simulink model "ekf2sim_example"  (R2014a)
settings: Solver=FixedStepDiscrete  StartTime=0  StopTime=200  RelTol=1e-3
settings Model: Creator=gcampa  LastModifiedBy=gcampa
settings DataIOCC: LimitDataPoints=off  SignalLoggingSaveFormat=ModelDataLogs  SaveOutput=off  SaveTime=off
settings OptimizationCC: BlockReduction=off  BooleanDataType=off  ExpressionDepthLimit=2147483647  InitFltsAndDblsToZero=on
settings DebuggingCC: SaveWithParameterizedLinksMsg=none  UnderspecifiedInitializationDetection=Classic  SignalResolutionControl=TryResolveAllWithWarning  SolverPrmCheckMsg=none  MultiTaskDSMMsg=warning  MultiTaskCondExecSysMsg=none  FcnCallInpInsideContextMsg=UseLocalSettings  StateNameClashWarn=warning
settings HardwareCC: TargetLongLongMode=on  TargetIntDivRoundTo=Zero  TargetEndianess=LittleEndian  TargetHWDeviceType=MATLAB Host  ProdEqTarget=off
settings RTWCC: IncludeERTFirstTime=on  RTWCompilerOptimization=On
settings GRTTargetCC: TargetFcnLib=ansi_tfl_tmw.mat  CombineOutputUpdateFcns=off  GRTInterface=on

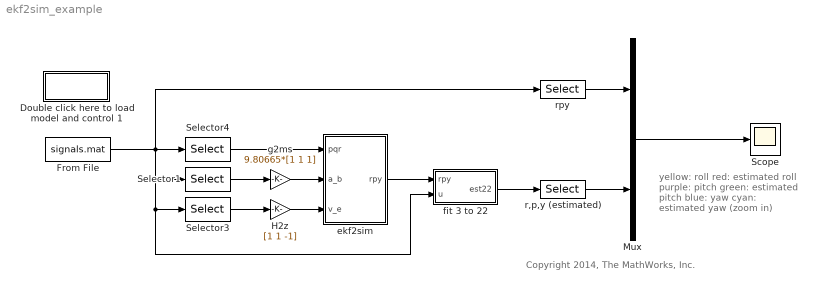
== system ekf2sim_example ==
  note: Copyright 2014, The MathWorks, Inc.
  note: yellow: roll
      | red: estimated roll
      | purple: pitch
      | green: estimated pitch
      | blue: yaw
      | cyan: estimated yaw
      | (zoom in)
  Double click here to load model and control 1 : Subsystem
      mask Display: disp('Measured \nSignals')
  From File : FromFile  FileName=signals.mat  SampleTime=0.05
  H2z : Gain  Gain=[1 1 -1]  SaturateOnIntegerOverflow=on  OutDataTypeStr=Inherit: Same as input  ParamDataTypeStr=Inherit: Same as input
  Mux : Mux  Inputs=[3 3]
  Scope : Scope
  Selector1 : Selector  InputPortWidth=22  Indices=16:18
  Selector3 : Selector  InputPortWidth=22  Indices=13:15
  Selector4 : Selector  InputPortWidth=22  Indices=[4:6]
  ekf2sim : Subsystem  mask(Attitude Estimator with 2-States EKF){W=diag([0.0723 0.1652]), V=diag([1 1e3]), v0=60*[cos(0) sin(0) sin(-0.0293682)], x0=[0 -0.0293682]', P0=zeros(2), Plim=0.01, T=0.05}
      mask prompts: W "W (state noise covariance)"; V "V (output noise covariance)"; v0 "v0 (velocity initial condition)"; x0 "x0 (roll and pitch initial condition)"; P0 "P0 (initial condition for P)"; Plim "P limiter"; T "Sample Time"
      mask help: This block estimates the attitude, that is the roll pitch and yaw angles, (radians, output vector) of a rigid body from the angular velocity (rad/s first input), the acceleration in body frame (m/s, second input), and the velocity in earth frame (meters, third input). See the help for more information.
      mask Help:
      | This block estimates the attitude, that is the roll pitch and yaw angles, (radians, output vector) of a rigid body from the angular velocity (rad/s first input), the acceleration in body frame (m/s, second input), and the velocity in earth frame (meters, third input). See the help for more information.
      | <p>
      | The body coordinate frame has x pointing forward, y pointing right, and z pointing down, while the earth frame is a local frame with x pointing north, y pointing east, and z pointing down.
      | <p>
      | The internal EKF has 2 just states, that is the roll and pitch estimates (see below for more info). The initial condition for these states and their covariance matrix is set respectively in x0 and P0, (third and fourth parameter), while the (2 by 2) covariance matrices of the state and output noises, W and V, are set as the first and second parameter respectively. The fifth parameter, P limiter, is a scalar that limits the norm of P to prevent it from growing too much. Finally v0 is the the initial condition for the velocity in earth frame, and T is the sample time.
      | <p>
      | As for the algorithm used in this block, the yaw angle is approximated with the heading angle, and roll and pitch are calculated comparing the derivative of the velocity in earth frame with the acceleration in body frame (see "Real-Time Attitude and Position Estimation for Small UAVs Using Low-Cost Sensors. Derek B. Kingston and Randal W. Beard").
      | A minimal 2-states EKF then uses the angular velocity information to smooth out the results. This allows for a very fast (albeit somewhat approximate) algorithm that can be executed on inexpensive hardware.
      | <p>
      | In this block, the algorithm is implemented in pure Simulink (look under the mask to see it). See the attached presentation and the files in the "Comparison" folder for other possible ways to implement this EKF, like S-Functions (in C and MATLAB), System objects, S-Function Builder, Legacy Code Tool, and the MATLAB function block (using both internal and external states).
  fit 3 to 22 : Subsystem
  g2ms : Gain  Gain=9.80665*[1 1 1]  SaturateOnIntegerOverflow=on  OutDataTypeStr=Inherit: Same as input  ParamDataTypeStr=Inherit: Same as input
  r,p,y (estimated) : Selector  InputPortWidth=22  Indices=[9 8 7]
  rpy : Selector  InputPortWidth=22  Indices=[9 8 7]
  wires:
  fit 3 to 22/1(est22) -> r,p,y (estimated)/1
  Selector3/1 -> H2z/1
  Selector1/1 -> g2ms/1
  g2ms/1 -> ekf2sim/2(a_b)
  Selector4/1 -> ekf2sim/1(pqr)
  From File/1 -> rpy/1, fit 3 to 22/2(u), Selector3/1, Selector1/1, Selector4/1
  ekf2sim/1(rpy) -> fit 3 to 22/1(rpy)
  H2z/1 -> ekf2sim/3(v_e)
  rpy/1 -> Mux/1
  r,p,y (estimated)/1 -> Mux/2
  Mux/1 -> Scope/1

== system ekf2sim_example/Double click here to load model and control 1 ==
  note: x:
      |
      | 01    v           (m/s)
      | 02    alpha    (rad)
      | 03    beta      (rad)
      | 04    p           (rad/s)
      | 05    q           (rad/s)
      | 06    r            (rad/s)
      | 07    psi         (rad)
      | 08    theta     (rad)
      | 09    phi        (rad)
      | 10    x           (m)
      | 11    y           (m)
      | 12    H          (m)
      |
      | x_dot (NED earth frame):
      |
      | 13    x_dot     (m/s)
      | 14    y_dot     (m/s)
      | 15    z_dot     (m/s)
      |
      | accelerations:
      |
      | 16    Ax     (g)
      | 17    Ay     (g)
      | 18    Az     (g)
      |
      | controls:
      |
      | 19    delta elevators    (rad)
      | 20    delta ailerons      (rad)
      | 21    delta rudder        (rad)
      | 22    throttle             (Fx, N)
  note: An aircraft model in closed loop with an inner and outer loop feedback
      | linearization control system was used to generate attitude (roll, pitch and yaw)
      | as well as all the other relevant signals
  note: More information on the aircraft model and controllers can be found here:
      | http://www.mathworks.com/matlabcentral/fileexchange/3019-airlib

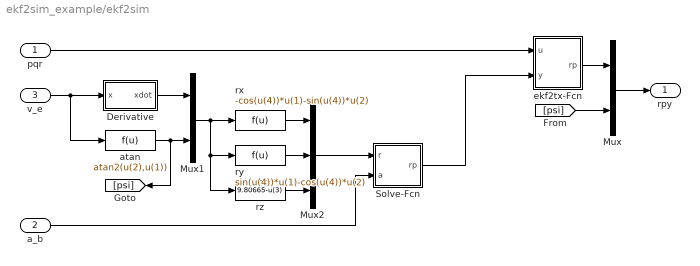
== system ekf2sim_example/ekf2sim ==
  pqr : Inport
  a_b : Inport  Port=2
  v_e : Inport  Port=3
  Derivative : Subsystem  mask(Time Derivative){T=T, x0=v0}
      mask prompts: T "Sampling Time"; x0 "Initial Condition"
      mask help: First order approximation of the time derivative of the input signal.
      mask Help: First order approximation of the time derivative of the input signal.
  Mux : Mux  Inputs=[2 1]
  Mux1 : Mux  Inputs=[3 1]
  Mux2 : Mux  Inputs=[1 1 1]
  Solve-Fcn : Subsystem
  atan : Fcn  Expr=atan2(u(2),u(1))  SampleTime=0.05
  ekf2tx-Fcn : Subsystem  mask(Extended Kalman Filter){W=W, V=V, x0=x0, P0=P0, Plim=Plim, T=T}
      mask prompts: Plim "P limiter"; T "Sample Time"
      mask help: Milimalistic 2-states Extended Kalman Filter for attitude estimation
  rx : Fcn  Expr=-cos(u(4))*u(1)-sin(u(4))*u(2)
  ry : Fcn  Expr=sin(u(4))*u(1)-cos(u(4))*u(2)
  rz : Fcn  Expr=9.80665-u(3)
  rpy : Outport
  wires:
  Mux/1 -> rpy/1
  pqr/1 -> ekf2tx-Fcn/1(u)
  a_b/1 -> Solve-Fcn/2(a)
  Solve-Fcn/1(rp) -> ekf2tx-Fcn/2(y)
  ekf2tx-Fcn/1(rp) -> Mux/1
  [psi] -> Mux/2
  Mux1/1 -> rz/1, ry/1, rx/1
  Derivative/1(xdot) -> Mux1/1
  atan/1 -> [psi], Mux1/2
  rx/1 -> Mux2/1
  ry/1 -> Mux2/2
  Mux2/1 -> Solve-Fcn/1(r)
  rz/1 -> Mux2/3
  v_e/1 -> Derivative/1(x), atan/1

== system ekf2sim_example/fit 3 to 22 ==
  rpy : Inport
  u : Inport  Port=2
  Mux : Mux  Inputs=[3 3 3 13]
  Selector1 : Selector  InputPortWidth=3  Indices=[3 2 1]
  Selector2 : Selector  InputPortWidth=22  Indices=13:15
  Selector3 : Selector  InputPortWidth=22  Indices=10:22
  Selector4 : Selector  InputPortWidth=22  Indices=4:6
  Vab(rpy,xyHdot) : Subsystem
  est22 : Outport
  wires:
  Selector3/1 -> Mux/4
  Mux/1 -> est22/1
  rpy/1 -> Selector1/1, Vab(rpy,xyHdot)/2(rpy)
  u/1 -> Selector4/1, Selector3/1, Selector2/1
  Selector4/1 -> Mux/2
  Vab(rpy,xyHdot)/1(vab) -> Mux/1
  Selector2/1 -> Vab(rpy,xyHdot)/1(xyHdot)
  Selector1/1 -> Mux/3

== system ekf2sim_example/ekf2sim/Derivative ==
  x : Inport  SampleTime=T
  Sum4 : Sum  Inputs=|+-  SaturateOnIntegerOverflow=on  InputSameDT=on  OutDataTypeStr=Inherit: Same as first input
  Unit Delay1 : UnitDelay  InitialCondition=x0  SampleTime=T
  gain : Gain  Gain=1/T  SampleTime=T  SaturateOnIntegerOverflow=on  OutDataTypeStr=Inherit: Same as input  ParamDataTypeStr=Inherit: Same as input
  xdot : Outport
  wires:
  gain/1 -> xdot/1
  x/1 -> Unit Delay1/1, Sum4/1
  Unit Delay1/1 -> Sum4/2
  Sum4/1 -> gain/1

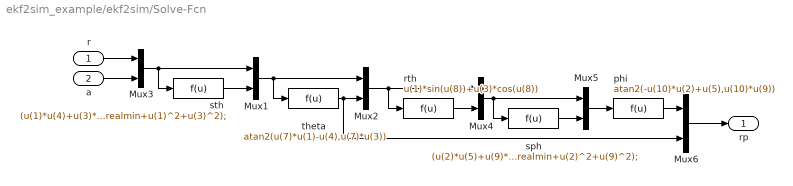
== system ekf2sim_example/ekf2sim/Solve-Fcn ==
  r : Inport
  a : Inport  Port=2
  Mux1 : Mux  Inputs=[6 1]
  Mux2 : Mux  Inputs=[7 1]
  Mux3 : Mux  Inputs=[3 3]
  Mux4 : Mux  Inputs=[8 1]
  Mux5 : Mux  Inputs=[9 1]
  Mux6 : Mux  Inputs=[1 1]
  phi : Fcn  Expr=atan2(-u(10)*u(2)+u(5),u(10)*u(9))
  rth : Fcn  Expr=u(1)*sin(u(8))+u(3)*cos(u(8))
  sph : Fcn  Expr=(u(2)*u(5)+u(9)*(abs(u(2)^2+u(9)^2-u(5)^2)^0.5))/(realmin+u(2)^2+u(9)^2);
  sth : Fcn  Expr=(u(1)*u(4)+u(3)*(abs(u(1)^2+u(3)^2-u(4)^2)^0.5))/(realmin+u(1)^2+u(3)^2);
  theta : Fcn  Expr=atan2(u(7)*u(1)-u(4),u(7)*u(3))
  rp : Outport
  wires:
  Mux6/1 -> rp/1
  phi/1 -> Mux6/1
  Mux5/1 -> phi/1
  sph/1 -> Mux5/2
  Mux4/1 -> Mux5/1, sph/1
  rth/1 -> Mux4/2
  Mux2/1 -> Mux4/1, rth/1
  theta/1 -> Mux6/2, Mux2/2
  Mux1/1 -> Mux2/1, theta/1
  sth/1 -> Mux1/2
  a/1 -> Mux3/2
  r/1 -> Mux3/1
  Mux3/1 -> Mux1/1, sth/1

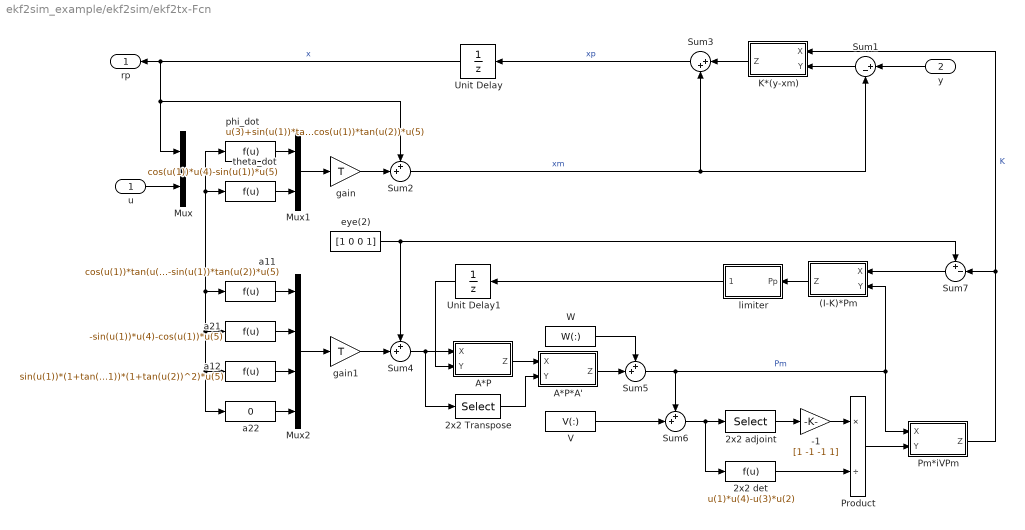
== system ekf2sim_example/ekf2sim/ekf2tx-Fcn ==
  u : Inport
  y : Inport  Port=2
  (I-K)*Pm : Subsystem  mask(2x2 Matrix Multiplication){}
      mask help:
      | Input 1   : elements of matrix X (2 by 2)
      |   Input 2   : elements of matrix Y (2 by 2)
      |   Output   : elements of matrix X*Y (2 by 2)
      mask Help:
      | <p>
      | Elements of input and output matrices are taken columnwise.
      | </p>
      mask Display: disp('Z=X*Y')
  -1 : Gain  Gain=[1 -1 -1 1]  SaturateOnIntegerOverflow=on  OutDataTypeStr=Inherit: Same as input  ParamDataTypeStr=Inherit: Same as input
  2x2 Transpose : Selector  InputPortWidth=4  Indices=[1 3 2 4]
  2x2 adjoint : Selector  InputPortWidth=4  Indices=[4 2 3 1]
  2x2 det : Fcn  Expr=u(1)*u(4)-u(3)*u(2)
  A*P : Subsystem  mask(2x2 Matrix Multiplication){}
      mask help:
      | Input 1   : elements of matrix X (2 by 2)
      |   Input 2   : elements of matrix Y (2 by 2)
      |   Output   : elements of matrix X*Y (2 by 2)
      mask Help:
      | <p>
      | Elements of input and output matrices are taken columnwise.
      | </p>
      mask Display: disp('Z=X*Y')
  A*P*A' : Subsystem  mask(2x2 Matrix Multiplication){}
      mask help:
      | Input 1   : elements of matrix X (2 by 2)
      |   Input 2   : elements of matrix Y (2 by 2)
      |   Output   : elements of matrix X*Y (2 by 2)
      mask Help:
      | <p>
      | Elements of input and output matrices are taken columnwise.
      | </p>
      mask Display: disp('Z=X*Y')
  K*(y-xm) : Subsystem  mask(2x2 Matrix Multiplication){}
      mask help:
      | Input 1   : elements of matrix X (2 by 2)
      |   Input 2   : elements of matrix Y (2 by 2)
      |   Output   : elements of matrix X*Y (2 by 2)
      mask Help:
      | <p>
      | Elements of input and output matrices are taken columnwise.
      | </p>
      mask Display: disp('Z=X*Y')
  Mux : Mux  Inputs=[2 3]
  Mux1 : Mux  Inputs=[1 1]
  Mux2 : Mux  Inputs=[1 1 1 1]
  Pm*iVPm : Subsystem  mask(2x2 Matrix Multiplication){}
      mask help:
      | Input 1   : elements of matrix X (2 by 2)
      |   Input 2   : elements of matrix Y (2 by 2)
      |   Output   : elements of matrix X*Y (2 by 2)
      mask Help:
      | <p>
      | Elements of input and output matrices are taken columnwise.
      | </p>
      mask Display: disp('Z=X*Y')
  Product : Product  Inputs=*/  RndMeth=Zero
  Sum1 : Sum  Inputs=|+-  SaturateOnIntegerOverflow=on  InputSameDT=on  OutDataTypeStr=Inherit: Same as first input
  Sum{2,4..6} (4 alike) : Sum  Inputs=++|  SaturateOnIntegerOverflow=on  InputSameDT=on  OutDataTypeStr=Inherit: Same as first input
  Sum3 : Sum  Inputs=|++  SaturateOnIntegerOverflow=on  InputSameDT=on  OutDataTypeStr=Inherit: Same as first input
  Sum7 : Sum  Inputs=+-|  SaturateOnIntegerOverflow=on  InputSameDT=on  OutDataTypeStr=Inherit: Same as first input
  Unit Delay : UnitDelay  InitialCondition=x0  SampleTime=T
  Unit Delay1 : UnitDelay  InitialCondition=P0(:)  SampleTime=T
  V : Constant  Value=V(:)
  W : Constant  Value=W(:)
  a11 : Fcn  Expr=cos(u(1))*tan(u(2))*u(4)-sin(u(1))*tan(u(2))*u(5)
  a12 : Fcn  Expr=sin(u(1))*(1+tan(u(2))^2)*u(4)+cos(u(1))*(1+tan(u(2))^2)*u(5)
  a21 : Fcn  Expr=-sin(u(1))*u(4)-cos(u(1))*u(5)
  a22 : Fcn  Expr=0
  eye(2) : Constant  Value=[1 0 0 1]
  gain : Gain  Gain=T  SaturateOnIntegerOverflow=on  OutDataTypeStr=Inherit: Same as input  ParamDataTypeStr=Inherit: Same as input
  gain1 : Gain  Gain=T  SampleTime=T  SaturateOnIntegerOverflow=on  OutDataTypeStr=Inherit: Same as input  ParamDataTypeStr=Inherit: Same as input
  limiter : Subsystem
  phi_dot : Fcn  Expr=u(3)+sin(u(1))*tan(u(2))*u(4)+cos(u(1))*tan(u(2))*u(5)
  theta_dot : Fcn  Expr=cos(u(1))*u(4)-sin(u(1))*u(5)
  rp : Outport
  wires:
  Sum2/1 -> Sum3/2, Sum1/2  "xm"
  gain/1 -> Sum2/2
  Mux1/1 -> gain/1
  phi_dot/1 -> Mux1/1
  theta_dot/1 -> Mux1/2
  Mux/1 -> phi_dot/1, theta_dot/1, a22/1, a12/1, a21/1, a11/1
  Unit Delay/1 -> Mux/1, Sum2/1, rp/1  "x"
  u/1 -> Mux/2
  y/1 -> Sum1/1
  Sum3/1 -> Unit Delay/1  "xp"
  a11/1 -> Mux2/1
  a21/1 -> Mux2/2
  a12/1 -> Mux2/3
  a22/1 -> Mux2/4
  Mux2/1 -> gain1/1
  gain1/1 -> Sum4/2
  eye(2)/1 -> Sum4/1, Sum7/1
  Sum4/1 -> A*P/1(X), 2x2 Transpose/1
  A*P/1(Z) -> A*P*A'/1(X)
  2x2 Transpose/1 -> A*P*A'/2(Y)
  Unit Delay1/1 -> A*P/2(Y)
  A*P*A'/1(Z) -> Sum5/2
  W/1 -> Sum5/1
  Sum5/1 -> Sum6/1, Pm*iVPm/1(X), (I-K)*Pm/2(Y)  "Pm"
  Sum6/1 -> 2x2 det/1, 2x2 adjoint/1
  2x2 adjoint/1 -> -1/1
  2x2 det/1 -> Product/2
  -1/1 -> Product/1
  Product/1 -> Pm*iVPm/2(Y)
  V/1 -> Sum6/2
  Pm*iVPm/1(Z) -> Sum7/2, K*(y-xm)/1(X)  "K"
  Sum7/1 -> (I-K)*Pm/1(X)
  K*(y-xm)/1(Z) -> Sum3/1
  Sum1/1 -> K*(y-xm)/2(Y)
  limiter/1(ball(Pp)) -> Unit Delay1/1
  (I-K)*Pm/1(Z) -> limiter/1(Pp)

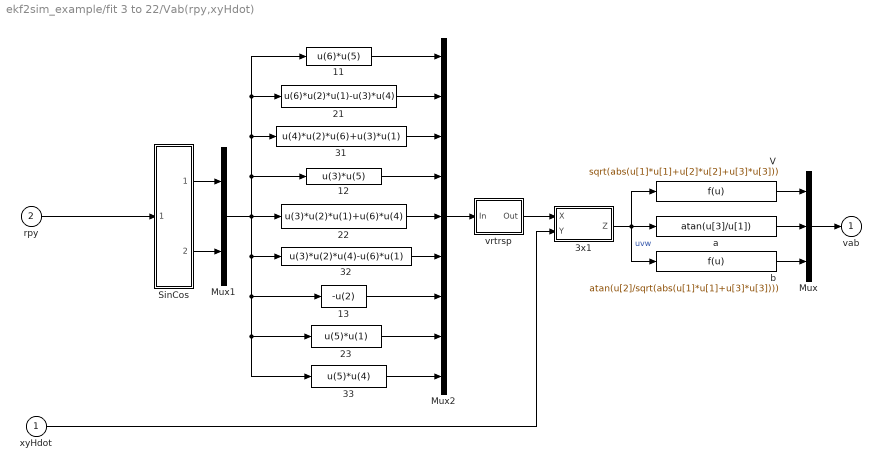
== system ekf2sim_example/fit 3 to 22/Vab(rpy,xyHdot) ==
  xyHdot : Inport
  rpy : Inport  Port=2
  11 : Fcn  Expr=u(6)*u(5)
  12 : Fcn  Expr=u(3)*u(5)
  13 : Fcn  Expr=-u(2)
  21 : Fcn  Expr=u(6)*u(2)*u(1)-u(3)*u(4)
  22 : Fcn  Expr=u(3)*u(2)*u(1)+u(6)*u(4)
  23 : Fcn  Expr=u(5)*u(1)
  31 : Fcn  Expr=u(4)*u(2)*u(6)+u(3)*u(1)
  32 : Fcn  Expr=u(3)*u(2)*u(4)-u(6)*u(1)
  33 : Fcn  Expr=u(5)*u(4)
  3x1 : Subsystem  mask(3x3 Matrix Multiplication){}
      mask help:
      | Input 1   : elements of matrix X (3 by 3)
      |   Input 2   : elements of matrix Y (3 by 3)
      |   Output   : elements of matrix X*Y (3 by 3)
      mask Help:
      | <p>
      | Elements of input and output matrices are taken columnwise.
      | </p>
      mask Display: disp('Z=X*Y')
  Mux : Mux  Inputs=3
  Mux1 : Mux  Inputs=2
  Mux2 : Mux  Inputs=9
  SinCos : Subsystem  mask(SinCos){}
      mask help: Compute the sine and cosine of input, u. u is in radians.
      mask Help: web(asbhelp);
      mask Display:
      | port_label('output',1,'sin(u)','texmode','on');
      | port_label('output',2,'cos(u)','texmode','on');
  V : Fcn  Expr=sqrt(abs(u[1]*u[1]+u[2]*u[2]+u[3]*u[3]))
  a : Fcn  Expr=atan(u[3]/u[1])
  b : Fcn  Expr=atan(u[2]/sqrt(abs(u[1]*u[1]+u[3]*u[3])))
  vrtrsp : Subsystem  mask(Simulink Matrix Library Block){dims=[3 3]}
      mask prompts: dims "[n m]"
      mask help:
      | Real Varying Matrix Transposition
      |   Input      : elements of matrix X (n by m)
      |   Output   : elements of matrix X' (m by n)
      mask Help:
      | <p>
      | Elements of input and output matrices are taken columnwise.
      | </p>
      | <p>
      | To use this block you should have the smxl library in your path.
      | </p>
      mask Display: disp('Y=X''')
  vab : Outport
  wires:
  rpy/1 -> SinCos/1(theta)
  3x1/1(Z) -> V/1, a/1, b/1  "uvw"
  Mux/1 -> vab/1
  a/1 -> Mux/2
  V/1 -> Mux/1
  b/1 -> Mux/3
  xyHdot/1 -> 3x1/2(Y)
  Mux2/1 -> vrtrsp/1(In)
  Mux1/1 -> 33/1, 23/1, 13/1, 32/1, 12/1, 31/1, 21/1, 11/1, 22/1
  SinCos/2(cos(theta)) -> Mux1/2
  SinCos/1(sin(theta)) -> Mux1/1
  11/1 -> Mux2/1
  21/1 -> Mux2/2
  31/1 -> Mux2/3
  12/1 -> Mux2/4
  22/1 -> Mux2/5
  32/1 -> Mux2/6
  13/1 -> Mux2/7
  23/1 -> Mux2/8
  33/1 -> Mux2/9
  vrtrsp/1(Out) -> 3x1/1(X)

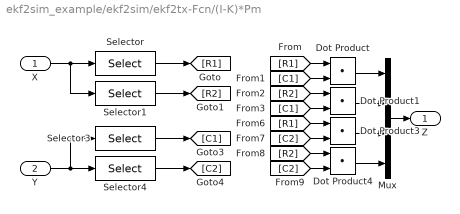
== system ekf2sim_example/ekf2sim/ekf2tx-Fcn/(I-K)*Pm ==
  X : Inport
  Y : Inport  Port=2
  Dot Product{,1,3..4} (4 alike) : DotProduct  InputSameDT=on  OutDataTypeStr=Inherit: Inherit via internal rule
  Mux : Mux  Inputs=ones(4,1)
  Selector : Selector  InputPortWidth=4  Indices=[1 3]
  Selector1 : Selector  InputPortWidth=4  Indices=[2 4]
  Selector3 : Selector  InputPortWidth=4  Indices=[1 2]
  Selector4 : Selector  InputPortWidth=4  Indices=[3 4]
  Z : Outport
  wires:
  Mux/1 -> Z/1
  Selector3/1 -> [C1]
  Selector4/1 -> [C2]
  Selector1/1 -> [R2]
  Y/1 -> Selector3/1, Selector4/1
  [C2] -> Dot Product4/2
  [R2] -> Dot Product4/1
  [C2] -> Dot Product3/2
  [R1] -> Dot Product3/1
  [C1] -> Dot Product1/2
  [R2] -> Dot Product1/1
  [C1] -> Dot Product/2
  [R1] -> Dot Product/1
  Selector/1 -> [R1]
  X/1 -> Selector/1, Selector1/1
  Dot Product/1 -> Mux/1
  Dot Product1/1 -> Mux/2
  Dot Product3/1 -> Mux/3
  Dot Product4/1 -> Mux/4

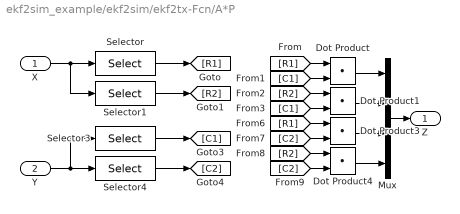
== system ekf2sim_example/ekf2sim/ekf2tx-Fcn/A*P ==
  X : Inport
  Y : Inport  Port=2
  Dot Product{,1,3..4} (4 alike) : DotProduct  InputSameDT=on  OutDataTypeStr=Inherit: Inherit via internal rule
  Mux : Mux  Inputs=ones(4,1)
  Selector : Selector  InputPortWidth=4  Indices=[1 3]
  Selector1 : Selector  InputPortWidth=4  Indices=[2 4]
  Selector3 : Selector  InputPortWidth=4  Indices=[1 2]
  Selector4 : Selector  InputPortWidth=4  Indices=[3 4]
  Z : Outport
  wires:
  Mux/1 -> Z/1
  Selector3/1 -> [C1]
  Selector1/1 -> [R2]
  Y/1 -> Selector3/1, Selector4/1
  [C2] -> Dot Product4/2
  [R2] -> Dot Product4/1
  [C2] -> Dot Product3/2
  [R1] -> Dot Product3/1
  [C1] -> Dot Product1/2
  [R2] -> Dot Product1/1
  [C1] -> Dot Product/2
  [R1] -> Dot Product/1
  Selector/1 -> [R1]
  X/1 -> Selector/1, Selector1/1
  Dot Product/1 -> Mux/1
  Dot Product1/1 -> Mux/2
  Dot Product3/1 -> Mux/3
  Dot Product4/1 -> Mux/4
  Selector4/1 -> [C2]

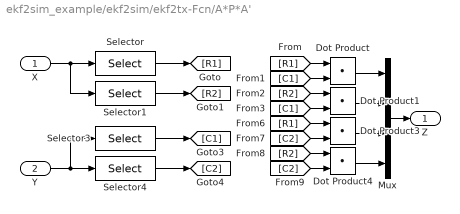
== system ekf2sim_example/ekf2sim/ekf2tx-Fcn/A*P*A' ==
  X : Inport
  Y : Inport  Port=2
  Dot Product{,1,3..4} (4 alike) : DotProduct  InputSameDT=on  OutDataTypeStr=Inherit: Inherit via internal rule
  Mux : Mux  Inputs=ones(4,1)
  Selector : Selector  InputPortWidth=4  Indices=[1 3]
  Selector1 : Selector  InputPortWidth=4  Indices=[2 4]
  Selector3 : Selector  InputPortWidth=4  Indices=[1 2]
  Selector4 : Selector  InputPortWidth=4  Indices=[3 4]
  Z : Outport
  wires:
  Dot Product4/1 -> Mux/4
  Dot Product3/1 -> Mux/3
  Dot Product1/1 -> Mux/2
  Dot Product/1 -> Mux/1
  X/1 -> Selector1/1, Selector/1
  Selector/1 -> [R1]
  [R1] -> Dot Product/1
  [C1] -> Dot Product/2
  [R2] -> Dot Product1/1
  [C1] -> Dot Product1/2
  [R1] -> Dot Product3/1
  [C2] -> Dot Product3/2
  [R2] -> Dot Product4/1
  [C2] -> Dot Product4/2
  Y/1 -> Selector4/1, Selector3/1
  Selector1/1 -> [R2]
  Selector4/1 -> [C2]
  Selector3/1 -> [C1]
  Mux/1 -> Z/1

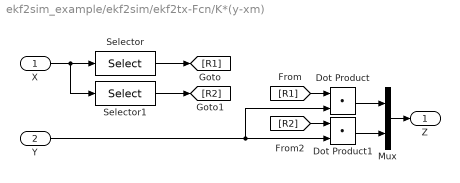
== system ekf2sim_example/ekf2sim/ekf2tx-Fcn/K*(y-xm) ==
  X : Inport
  Y : Inport  Port=2
  Dot Product : DotProduct  InputSameDT=on  OutDataTypeStr=Inherit: Inherit via internal rule
  Dot Product1 : DotProduct  InputSameDT=on  OutDataTypeStr=Inherit: Inherit via internal rule
  Mux : Mux  Inputs=ones(2,1)
  Selector : Selector  InputPortWidth=4  Indices=[1 3]
  Selector1 : Selector  InputPortWidth=4  Indices=[2 4]
  Z : Outport
  wires:
  Dot Product1/1 -> Mux/2
  Dot Product/1 -> Mux/1
  X/1 -> Selector1/1, Selector/1
  Selector/1 -> [R1]
  [R1] -> Dot Product/1
  [R2] -> Dot Product1/1
  Y/1 -> Dot Product1/2, Dot Product/2
  Selector1/1 -> [R2]
  Mux/1 -> Z/1

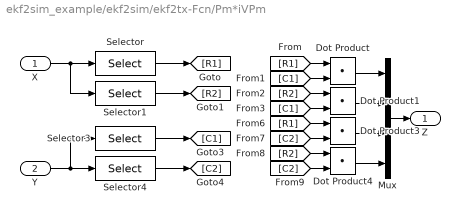
== system ekf2sim_example/ekf2sim/ekf2tx-Fcn/Pm*iVPm ==
  X : Inport
  Y : Inport  Port=2
  Dot Product{,1,3..4} (4 alike) : DotProduct  InputSameDT=on  OutDataTypeStr=Inherit: Inherit via internal rule
  Mux : Mux  Inputs=ones(4,1)
  Selector : Selector  InputPortWidth=4  Indices=[1 3]
  Selector1 : Selector  InputPortWidth=4  Indices=[2 4]
  Selector3 : Selector  InputPortWidth=4  Indices=[1 2]
  Selector4 : Selector  InputPortWidth=4  Indices=[3 4]
  Z : Outport
  wires:
  Mux/1 -> Z/1
  Selector3/1 -> [C1]
  Selector4/1 -> [C2]
  Selector1/1 -> [R2]
  Y/1 -> Selector3/1, Selector4/1
  [C2] -> Dot Product4/2
  [R2] -> Dot Product4/1
  [C2] -> Dot Product3/2
  [R1] -> Dot Product3/1
  [C1] -> Dot Product1/2
  [R2] -> Dot Product1/1
  [C1] -> Dot Product/2
  [R1] -> Dot Product/1
  Selector/1 -> [R1]
  X/1 -> Selector/1, Selector1/1
  Dot Product/1 -> Mux/1
  Dot Product1/1 -> Mux/2
  Dot Product3/1 -> Mux/3
  Dot Product4/1 -> Mux/4

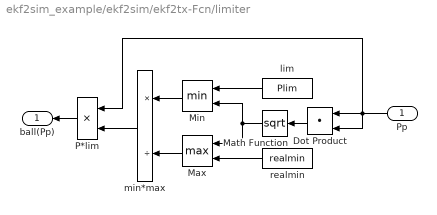
== system ekf2sim_example/ekf2sim/ekf2tx-Fcn/limiter ==
  Pp : Inport
  Dot Product : DotProduct  InputSameDT=on  OutDataTypeStr=Inherit: Inherit via internal rule
  Math Function : Math  Operator=sqrt  SaturateOnIntegerOverflow=on
  Max : MinMax  Function=max  Inputs=2
  Min : MinMax  Inputs=2
  P*lim : Product  Inputs=**  RndMeth=Zero
  lim : Constant  Value=Plim
  min*max : Product  Inputs=*/  RndMeth=Zero
  realmin : Constant  Value=realmin
  ball(Pp) : Outport
  wires:
  Pp/1 -> Dot Product/1, Dot Product/2, P*lim/1
  Dot Product/1 -> Math Function/1
  Math Function/1 -> Max/1, Min/2
  P*lim/1 -> ball(Pp)/1
  realmin/1 -> Max/2
  lim/1 -> Min/1
  Min/1 -> min*max/1
  Max/1 -> min*max/2
  min*max/1 -> P*lim/2

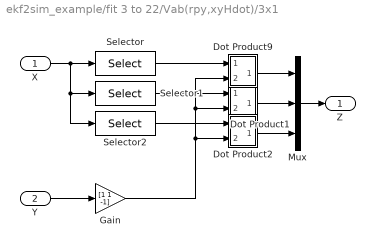
== system ekf2sim_example/fit 3 to 22/Vab(rpy,xyHdot)/3x1 ==
  X : Inport
  Y : Inport  Port=2
  Dot Product1 : Subsystem  mask(Dot Product){}
      mask help:
      | Inner (dot) product.
      | y = sum(conj(u1).*u2). The operand u1 corresponds to the top (or left) input port.
      mask init:
      | t=(0:.1:2*pi)';
      | x=cos(t);
      | y=sin(t);
      | r=0.05;
      mask Help: Computes the inner (dot) product of the inputs: sum(u1.*u2).  The inputs are vectors of the same length. Output is a scalar.
      mask Display: patch([x*r+0.5],[y*r+0.5])
  Dot Product2 : Subsystem  mask(Dot Product){}
      mask help:
      | Inner (dot) product.
      | y = sum(conj(u1).*u2). The operand u1 corresponds to the top (or left) input port.
      mask init:
      | t=(0:.1:2*pi)';
      | x=cos(t);
      | y=sin(t);
      | r=0.05;
      mask Help: Computes the inner (dot) product of the inputs: sum(u1.*u2).  The inputs are vectors of the same length. Output is a scalar.
      mask Display: patch([x*r+0.5],[y*r+0.5])
  Dot Product9 : Subsystem  mask(Dot Product){}
      mask help:
      | Inner (dot) product.
      | y = sum(conj(u1).*u2). The operand u1 corresponds to the top (or left) input port.
      mask init:
      | t=(0:.1:2*pi)';
      | x=cos(t);
      | y=sin(t);
      | r=0.05;
      mask Help: Computes the inner (dot) product of the inputs: sum(u1.*u2).  The inputs are vectors of the same length. Output is a scalar.
      mask Display: patch([x*r+0.5],[y*r+0.5])
  Gain : Gain  Gain=[1 1 -1]  OutDataTypeStr=Inherit: Same as input  ParamDataTypeStr=Inherit: Same as input
  Mux : Mux  Inputs=3
  Selector : Selector  InputPortWidth=9  Indices=[1:3]
  Selector1 : Selector  InputPortWidth=9  Indices=[4:6]
  Selector2 : Selector  InputPortWidth=9  Indices=[7:9]
  Z : Outport
  wires:
  X/1 -> Selector/1, Selector1/1, Selector2/1
  Selector/1 -> Dot Product9/1(In1)
  Dot Product9/1(Out1) -> Mux/1
  Dot Product1/1(Out1) -> Mux/2
  Selector1/1 -> Dot Product1/1(In1)
  Selector2/1 -> Dot Product2/1(In1)
  Dot Product2/1(Out1) -> Mux/3
  Y/1 -> Gain/1
  Gain/1 -> Dot Product2/2(In2), Dot Product1/2(In2), Dot Product9/2(In2)
  Mux/1 -> Z/1

== system ekf2sim_example/fit 3 to 22/Vab(rpy,xyHdot)/SinCos ==
  theta : Inport
  cosine : Trigonometry  Operator=cos
  sine : Trigonometry
  sin(theta) : Outport
  cos(theta) : Outport  Port=2
  wires:
  theta/1 -> sine/1, cosine/1
  sine/1 -> sin(theta)/1
  cosine/1 -> cos(theta)/1

== system ekf2sim_example/fit 3 to 22/Vab(rpy,xyHdot)/vrtrsp ==
  In : Inport
  Selector : Selector  InputPortWidth=dims(1)*dims(2)  Indices=reshape(reshape(1:dims(1)*dims(2),dims(1),dims(2))',dims(1)*dims(2),1)
  Out : Outport
  wires:
  Selector/1 -> Out/1
  In/1 -> Selector/1

== system ekf2sim_example/fit 3 to 22/Vab(rpy,xyHdot)/3x1/Dot Product1 ==
  In1 : Inport
  In2 : Inport  Port=2
  S-Function : S-Function  FunctionName=sdotproduct  EnableBusSupport=off
  Out1 : Outport
  wires:
  S-Function/1 -> Out1/1
  In1/1 -> S-Function/1
  In2/1 -> S-Function/2

== system ekf2sim_example/fit 3 to 22/Vab(rpy,xyHdot)/3x1/Dot Product2 ==
  In1 : Inport
  In2 : Inport  Port=2
  S-Function : S-Function  FunctionName=sdotproduct  EnableBusSupport=off
  Out1 : Outport
  wires:
  In2/1 -> S-Function/2
  In1/1 -> S-Function/1
  S-Function/1 -> Out1/1

== system ekf2sim_example/fit 3 to 22/Vab(rpy,xyHdot)/3x1/Dot Product9 ==
  In1 : Inport
  In2 : Inport  Port=2
  S-Function : S-Function  FunctionName=sdotproduct  EnableBusSupport=off
  Out1 : Outport
  wires:
  In2/1 -> S-Function/2
  In1/1 -> S-Function/1
  S-Function/1 -> Out1/1
